simulink subsystem "s_pacemaker_stateflow"  (R2024b)
settings: Solver=VariableStepAuto  StartTime=0.0  StopTime=10.0  RelTol=1e-3
settings Model: Creator=marwa  LastModifiedBy=habel

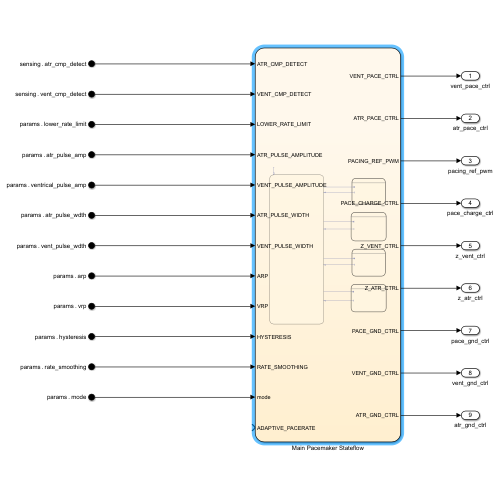
[thumbnail: Simulink's stored preview of the top-level diagram]
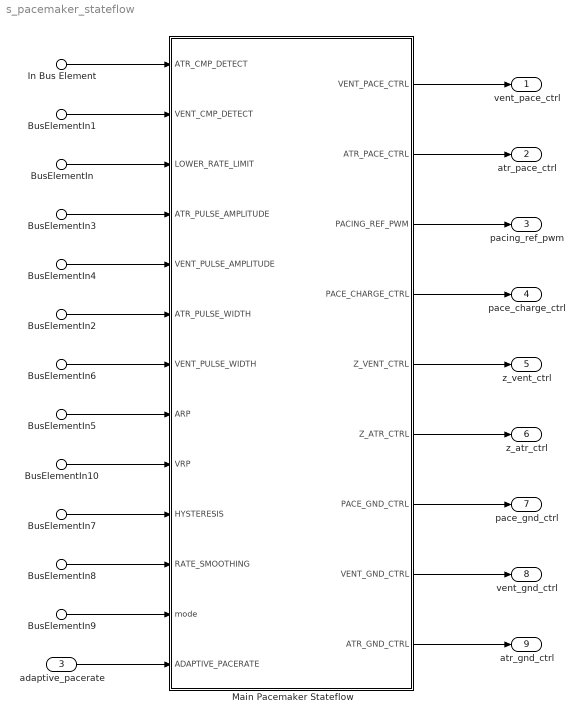
== system s_pacemaker_stateflow ==
  BusElementIn5 : Inport  PortName=params  Element=arp
  BusElementIn : Inport  PortName=params  Element=lower_rate_limit
  BusElementIn2 : Inport  PortName=params  Element=atr_pulse_wdth
  BusElementIn3 : Inport  PortName=params  Element=atr_pulse_amp
  BusElementIn4 : Inport  PortName=params  Element=vent_pulse_amp
  BusElementIn6 : Inport  PortName=params  Element=vent_pulse_wdth
  BusElementIn7 : Inport  PortName=params  Element=hysteresis
  BusElementIn8 : Inport  PortName=params  Element=rate_smoothing
  BusElementIn9 : Inport  PortName=params  Element=mode
  BusElementIn10 : Inport  PortName=params  Element=vrp
  In Bus Element : Inport  Port=2  PortName=sensing  Element=atr_cmp_detect
  BusElementIn1 : Inport  Port=2  PortName=sensing  Element=vent_cmp_detect
  adaptive_pacerate : Inport  Port=3
  Main Pacemaker Stateflow : Stateflow chart  TreatAsAtomicUnit=on
      settings: PortSchema="{\"entries\":[{\"content\":{\"sides\":[{\"content\":{\"connectorIds\":[\"In1\",\"In2\",\"In3\",\"In6\",\"In4\",\"In7\",\"In5\",\"In8\",\"In9\",\"In10\",\"In11\",\"In12\",\"In13\"]},\"type\":\"ConnectorPlacement.EquallySpacedRectSide\",\"uuid\":\"e04c6c9d-b568-4760-aae3-37103fc4b8a5\"},{\"content\":{\"connectorIds\":[\"Out1\",\"Out2\",\"Out3\",\"Out4\",\"Out5\",\"Out6\",\"Out7\",\"Out8\",\"Out9\"],\"side\":\"RIGHT\"},\"type\":\"ConnectorPlacement.EquallySpacedRectSide\",\"uuid\":\"410f5465-af00-4611-9887-c67099d36fd9\"},{\"content\":{\"connectorIds\":[],\"side\":\"TOP\"},\"type\":\"ConnectorPlacement.EquallySpacedRectSide\",\"uuid\":\"117107fa-ec70-4a57-9ea7-207f77d687e8\"}]},\"type\":\"ConnectorPlacement.EquallySpacedConnector\",\"uuid\":\"376840e9-6019-4e50-8c40-c1322fd1edca\"}],\"packageUris\":[\"http://schema.mathworks.com/mf0/Connector/19700101\"],\"version\":\"1.0\"}"
  vent_pace_ctrl : Outport
  atr_pace_ctrl : Outport  Port=2
  pacing_ref_pwm : Outport  Port=3
  pace_charge_ctrl : Outport  Port=4
  z_vent_ctrl : Outport  Port=5
  z_atr_ctrl : Outport  Port=6
  pace_gnd_ctrl : Outport  Port=7
  vent_gnd_ctrl : Outport  Port=8
  atr_gnd_ctrl : Outport  Port=9
  wires:
  BusElementIn/1 -> Main Pacemaker Stateflow/3(LOWER_RATE_LIMIT)
  BusElementIn2/1 -> Main Pacemaker Stateflow/7(ATR_PULSE_WIDTH)
  BusElementIn3/1 -> Main Pacemaker Stateflow/6(ATR_PULSE_AMPLITUDE)
  BusElementIn4/1 -> Main Pacemaker Stateflow/4(VENT_PULSE_AMPLITUDE)
  BusElementIn5/1 -> Main Pacemaker Stateflow/8(ARP)
  BusElementIn10/1 -> Main Pacemaker Stateflow/9(VRP)
  BusElementIn9/1 -> Main Pacemaker Stateflow/12(mode)
  BusElementIn7/1 -> Main Pacemaker Stateflow/10(HYSTERESIS)
  BusElementIn8/1 -> Main Pacemaker Stateflow/11(RATE_SMOOTHING)
  BusElementIn6/1 -> Main Pacemaker Stateflow/5(VENT_PULSE_WIDTH)
  In Bus Element/1 -> Main Pacemaker Stateflow/1(ATR_CMP_DETECT)
  BusElementIn1/1 -> Main Pacemaker Stateflow/2(VENT_CMP_DETECT)
  Main Pacemaker Stateflow/1(VENT_PACE_CTRL) -> vent_pace_ctrl/1
  Main Pacemaker Stateflow/2(ATR_PACE_CTRL) -> atr_pace_ctrl/1
  Main Pacemaker Stateflow/3(PACING_REF_PWM) -> pacing_ref_pwm/1
  Main Pacemaker Stateflow/4(PACE_CHARGE_CTRL) -> pace_charge_ctrl/1
  Main Pacemaker Stateflow/5(Z_VENT_CTRL) -> z_vent_ctrl/1
  Main Pacemaker Stateflow/6(Z_ATR_CTRL) -> z_atr_ctrl/1
  Main Pacemaker Stateflow/7(PACE_GND_CTRL) -> pace_gnd_ctrl/1
  Main Pacemaker Stateflow/8(VENT_GND_CTRL) -> vent_gnd_ctrl/1
  Main Pacemaker Stateflow/9(ATR_GND_CTRL) -> atr_gnd_ctrl/1
  adaptive_pacerate/1 -> Main Pacemaker Stateflow/13(ADAPTIVE_PACERATE)

== stateflow chart s_pacemaker_stateflow/Main Pacemaker Stateflow ==
  state Startup
  state AOO
    state CHARGING
      entry:
      %% Charging C22 (to deliver pulse)
      ATR_PACE_CTRL= 0;
      VENT_PACE_CTRL = 0;
      PACING_REF_PWM = ATR_PULSE_AMPLITUDE;
      PACE_CHARGE_CTRL = 1;
      %% Discharging C21 (ensure net current flow is 0)
      PACE_GND_CTRL = 1;
      VENT_PACE_CTRL = 0;
      Z_ATR_CTRL = 0;
      Z_VENT_CTRL = 0;
      ATR_GND_CTRL = 1;
      VENT_GND_CTRL = 0;
    state PACING
      %% Discharge pulse
      entry:
      PACE_CHARGE_CTRL = 0;
      PACE_GND_CTRL = 1;
      ATR_PACE_CTRL = 1;
      ATR_GND_CTRL = 0;
      Z_ATR_CTRL = 0;
      Z_VENT_CTRL = 0;
      VENT_GND_CTRL = 0;
      VENT_PACE_CTRL = 0;
    AOO.CHARGING -> AOO.PACING [order 1] : %%Pace Ready - when interval for one pulse is completed
        | [after(1/(double(LOWER_RATE_LIMIT)/60000) - double(ATR_PULSE_WIDTH), msec)]
    AOO.PACING -> AOO.CHARGING : %%Recharge Ready - after atrium pulse finishes
        | [after(ATR_PULSE_WIDTH, msec)]
  state AAI
    state CHARGING
      entry:
      %%Charging C22 (to deliver pulse)
      ATR_PACE_CTRL = 0;
      VENT_PACE_CTRL = 0;
      PACE_CHARGE_CTRL = 1;
      %%Discharging Blocking Cap (C21) - net current 0
      PACE_GND_CTRL = 1;
      Z_ATR_CTRL = 0;
      Z_VENT_CTRL = 0;
      ATR_GND_CTRL = 1;
      VENT_GND_CTRL = 0;
      PACING_REF_PWM = ATR_PULSE_AMPLITUDE;
    state PACING
      %%Deliver pulse
      entry:
      PACE_CHARGE_CTRL = 0;
      PACE_GND_CTRL = 1;
      ATR_PACE_CTRL = 1;
      ATR_GND_CTRL = 0;
      Z_ATR_CTRL = 0;
      Z_VENT_CTRL = 0;
      VENT_GND_CTRL = 0;
      VENT_PACE_CTRL = 0;
    AAI.CHARGING -> (junction 142) [order 1] : %%After refractory period, consider delivering pulse
        | [after(ARP, msec)]
    (junction 142) -> AAI.PACING [order 1] : %%Pace Ready - after no detection of intrinsic heart-rate and after atrial refractory period
        | [after(1/(double(LOWER_RATE_LIMIT)/60000) - double(ATR_PULSE_WIDTH) - ARP, msec) && ATR_CMP_DETECT == false]
    (junction 142) -> AAI.CHARGING [order 2] : %%Inhibit pacing if natural heart-rate detected
        | [ATR_CMP_DETECT == true]
    AAI.PACING -> AAI.CHARGING : %%Recharge Ready - after atrium pulse completes
        | [after(ATR_PULSE_WIDTH, msec)]
  state VOO
    state CHARGING
      entry:
      %% Charging C22 (to deliver pulse)
      ATR_PACE_CTRL= 0;
      VENT_PACE_CTRL = 0;
      PACING_REF_PWM = VENT_PULSE_AMPLITUDE;
      PACE_CHARGE_CTRL = 1;
      %% Discharging C21 (ensure net current is 0)
      PACE_GND_CTRL = 1;
      VENT_PACE_CTRL = 0;
      Z_ATR_CTRL = 0;
      Z_VENT_CTRL = 0;
      ATR_GND_CTRL = 0;
      VENT_GND_CTRL = 1;
    state PACING
      %%Deliver pulse
      entry:
      PACE_CHARGE_CTRL = 0;
      PACE_GND_CTRL = 1;
      ATR_PACE_CTRL = 0;
      ATR_GND_CTRL = 0;
      Z_ATR_CTRL = 0;
      Z_VENT_CTRL = 0;
      VENT_GND_CTRL = 0;
      VENT_PACE_CTRL = 1;
    VOO.CHARGING -> VOO.PACING [order 2] : %%Pace Ready - after interval for one pulse is completed
        | [after(60000/(double(LOWER_RATE_LIMIT)) - double(VENT_PULSE_WIDTH), msec)]
    VOO.PACING -> VOO.CHARGING : %%Recharge Ready - when ventricular pulse time finishes
        | [after(VENT_PULSE_WIDTH, msec)]
  state VVI
    state CHARGING
      entry:
      %%Charging C22
      ATR_PACE_CTRL = 0;
      VENT_PACE_CTRL = 0;
      PACE_CHARGE_CTRL = 1;
      %%Discharging Blocking Cap
      PACE_GND_CTRL = 1;
      Z_ATR_CTRL = 0;
      Z_VENT_CTRL = 0;
      ATR_GND_CTRL = 0;
      VENT_GND_CTRL = 1;
      PACING_REF_PWM = VENT_PULSE_AMPLITUDE;
    state PACING
      entry:
      PACE_CHARGE_CTRL = 0;
      PACE_GND_CTRL = 1;
      ATR_PACE_CTRL = 0;
      ATR_GND_CTRL = 0;
      Z_ATR_CTRL = 0;
      Z_VENT_CTRL = 0;
      VENT_GND_CTRL = 0;
      VENT_PACE_CTRL = 1;
    VVI.CHARGING -> (junction 128) [order 1] : %%After refractory period is complete, consider delivering pulse
        | [after(VRP, msec)]
    (junction 128) -> VVI.PACING [order 1] : %%Pace Ready - after no detection of intrinsic heart-rate, and ventricular refractory period is complete
        | [after(1/(double(LOWER_RATE_LIMIT)/60000) - double(VENT_PULSE_WIDTH) - VRP, msec) && VENT_CMP_DETECT == false]
    (junction 128) -> VVI.CHARGING [order 2] : %% Inhibit pulse if intrinsic heart-rate is detected
        | [VENT_CMP_DETECT == true]
    VVI.PACING -> VVI.CHARGING : %%Recharge - after ventricular pulse is finished
        | [after(VENT_PULSE_WIDTH, msec)]
  state AOOR
    state CHARGING
      entry:
      %% Charging C22 (to deliver pulse)
      ATR_PACE_CTRL= 0;
      VENT_PACE_CTRL = 0;
      PACING_REF_PWM = ATR_PULSE_AMPLITUDE;
      PACE_CHARGE_CTRL = 1;
      %% Discharging C21 (ensure net current is 0)
      PACE_GND_CTRL = 1;
      VENT_PACE_CTRL = 0;
      Z_ATR_CTRL = 0;
      Z_VENT_CTRL = 0;
      ATR_GND_CTRL = 1;
      VENT_GND_CTRL = 0;
    state PACING
      %%Deliver pulse
      entry:
      PACE_CHARGE_CTRL = 0;
      PACE_GND_CTRL = 1;
      ATR_PACE_CTRL = 1;
      ATR_GND_CTRL = 0;
      Z_ATR_CTRL = 0;
      Z_VENT_CTRL = 0;
      VENT_GND_CTRL = 0;
      VENT_PACE_CTRL = 0;
    AOOR.CHARGING -> AOOR.PACING [order 1] : %%Pace Ready - After the dynamic interval for one pulse
        | [after(60000/(double(ADAPTIVE_PACERATE)), msec)]
    AOOR.PACING -> AOOR.CHARGING : %%Recharge Ready - after atrial pulse finishes
        | [after(ATR_PULSE_WIDTH, msec)]
  state VOOR
    state CHARGING
      entry:
      %% Charging C22 (to deliver pulse)
      ATR_PACE_CTRL= 0;
      VENT_PACE_CTRL = 0;
      PACING_REF_PWM = VENT_PULSE_AMPLITUDE;
      PACE_CHARGE_CTRL = 1;
      %% Discharging C21 (ensure net current is 0)
      PACE_GND_CTRL = 1;
      VENT_PACE_CTRL = 0;
      Z_ATR_CTRL = 0;
      Z_VENT_CTRL = 0;
      ATR_GND_CTRL = 0;
      VENT_GND_CTRL = 1;
    state PACING
      %% Deliver pulse
      entry:
      PACE_CHARGE_CTRL = 0;
      PACE_GND_CTRL = 1;
      ATR_PACE_CTRL = 0;
      ATR_GND_CTRL = 0;
      Z_ATR_CTRL = 0;
      Z_VENT_CTRL = 0;
      VENT_GND_CTRL = 0;
      VENT_PACE_CTRL = 1;
    VOOR.CHARGING -> VOOR.PACING [order 2] : %%Pace Ready - after dynamic interval for pulse
        | [after(60000/(double(ADAPTIVE_PACERATE)), msec)]
    VOOR.PACING -> VOOR.CHARGING : %%Recharge Ready - after ventricular pulse finishes
        | [after(VENT_PULSE_WIDTH, msec)]
  state AAIR
    state CHARGING
      entry:
      %%Charging C22 (to deliver pulse)
      ATR_PACE_CTRL = 0;
      VENT_PACE_CTRL = 0;
      PACE_CHARGE_CTRL = 1;
      %%Discharging Blocking Cap (C21) (net current 0)
      PACE_GND_CTRL = 1;
      Z_ATR_CTRL = 0;
      Z_VENT_CTRL = 0;
      ATR_GND_CTRL = 1;
      VENT_GND_CTRL = 0;
      PACING_REF_PWM = ATR_PULSE_AMPLITUDE;
    state PACING
      %%Deliver pulse
      entry:
      PACE_CHARGE_CTRL = 0;
      PACE_GND_CTRL = 1;
      ATR_PACE_CTRL = 1;
      ATR_GND_CTRL = 0;
      Z_ATR_CTRL = 0;
      Z_VENT_CTRL = 0;
      VENT_GND_CTRL = 0;
      VENT_PACE_CTRL = 0;
    AAIR.CHARGING -> (junction 284) [order 1] : %%After refractory period, consider delivering pulse
        | [after(ARP, msec)]
    (junction 284) -> AAIR.PACING [order 1] : %%Pace Ready - same as AAI but using dynamic interval
        | [after(1/(double(ADAPTIVE_PACERATE)/60000) - double(ATR_PULSE_WIDTH) - ARP, msec) && ATR_CMP_DETECT == false]
    (junction 284) -> AAIR.CHARGING [order 2] : %%if intrinsic heart-rate detected, inhibit response
        | [ATR_CMP_DETECT == true]
    AAIR.PACING -> AAIR.CHARGING : %%Recharge Ready - after atrial pulse completes
        | [after(ATR_PULSE_WIDTH, msec)]
  state VVIR
    state CHARGING
      entry:
      %%Charging C22 (to deliver pulse)
      ATR_PACE_CTRL = 0;
      VENT_PACE_CTRL = 0;
      PACE_CHARGE_CTRL = 1;
      %%Discharging Blocking Cap C21 (net current is 0)
      PACE_GND_CTRL = 1;
      Z_ATR_CTRL = 0;
      Z_VENT_CTRL = 0;
      ATR_GND_CTRL = 0;
      VENT_GND_CTRL = 1;
      PACING_REF_PWM = VENT_PULSE_AMPLITUDE;
    state PACING
      %%deliver pulse
      entry:
      PACE_CHARGE_CTRL = 0;
      PACE_GND_CTRL = 1;
      ATR_PACE_CTRL = 0;
      ATR_GND_CTRL = 0;
      Z_ATR_CTRL = 0;
      Z_VENT_CTRL = 0;
      VENT_GND_CTRL = 0;
      VENT_PACE_CTRL = 1;
    (junction 273) -> VVIR.PACING [order 1] : %%Pace Ready - same as VVI but using dynamic interval
        | [after(1/(double(ADAPTIVE_PACERATE)/60000) - double(VENT_PULSE_WIDTH) - VRP, msec) && VENT_CMP_DETECT == false]
    (junction 273) -> VVIR.CHARGING [order 2] : %% if intrinsic heart-rate detected, inhibit response
        | [VENT_CMP_DETECT == true]
    VVIR.CHARGING -> (junction 273) [order 1] : %%After refractory period, consider delivering pulse
        | [after(VRP, msec)]
    VVIR.PACING -> VVIR.CHARGING : %%Recharge - After ventricular pulse is complete
        | [after(VENT_PULSE_WIDTH, msec)]
  Startup -> AAIR.CHARGING [order 3] : [mode == 7]
  AAIR.CHARGING -> Startup [order 2] : [mode ~= 7]
  Startup -> VVIR.CHARGING [order 2] : [mode == 8]
  Startup -> AOOR.CHARGING [order 7] : [mode == 5]
  Startup -> VOOR.CHARGING [order 8] : [mode == 6]
  Startup -> VOO.CHARGING [order 5] : [mode == 3]
  Startup -> VVI.CHARGING [order 6] : [mode == 4]
  AAI.CHARGING -> Startup [order 2] : [mode ~= 2]
  VVIR.CHARGING -> Startup [order 2] : [mode ~= 8]
  AOO.CHARGING -> Startup [order 2] : [mode ~= 1]
  AOOR.CHARGING -> Startup [order 2] : [mode ~= 5]
  VVI.CHARGING -> Startup [order 2] : [mode ~= 4]
  Startup -> AOO.CHARGING [order 1] : [mode == 1]
  VOOR.CHARGING -> Startup [order 1] : [mode ~= 6]
  VOO.CHARGING -> Startup [order 1] : [mode ~= 3]
  (default) -> Startup
  Startup -> AAI.CHARGING [order 4] : [mode == 2]
  data: ATR_CMP_DETECT input; VENT_CMP_DETECT input; VENT_PACE_CTRL output; ATR_PACE_CTRL output; PACING_REF_PWM output; PACE_CHARGE_CTRL output; Z_VENT_CTRL output; Z_ATR_CTRL output; PACE_GND_CTRL output; VENT_GND_CTRL output; ATR_GND_CTRL output; LOWER_RATE_LIMIT input; VENT_PULSE_AMPLITUDE input; VENT_PULSE_WIDTH input; ATR_PULSE_AMPLITUDE input; ATR_PULSE_WIDTH input; ARP input; VRP input; HYSTERESIS input; RATE_SMOOTHING input; mode input; ADAPTIVE_PACERATE input
